simulink model "Project2"  (R2025b)
settings: Solver=VariableStepAuto  StartTime=0.0  StopTime=10  RelTol=1e-3
libraries: simulink x1
settings Model: Creator=night  LastModifiedBy=night

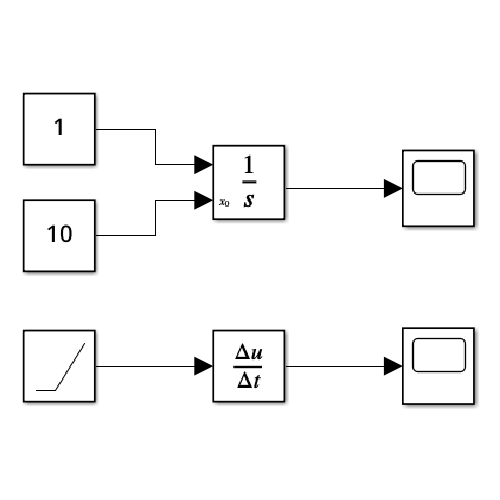
[thumbnail: Simulink's stored preview of the top-level diagram]
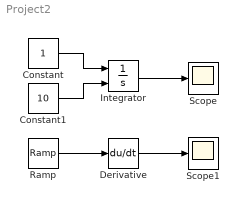
== system Project2 ==
  Constant : Constant
  Constant1 : Constant  Value=10
  Derivative : Derivative
  Integrator : Integrator  InitialConditionSource=external  InitialCondition=10
  Ramp : simulink/Sources/Ramp  slope=1  start=0  InitialOutput=0
  Scope : Scope
      settings: ActiveDisplayYMinimum=8.7500000000000036  ActiveDisplayYMaximum=21.249999999999964
  Scope1 : Scope
      settings: ActiveDisplayYMinimum=-0.12499999999999997  ActiveDisplayYMaximum=1.125
  wires:
  Constant/1 -> Integrator/1
  Integrator/1 -> Scope/1
  Derivative/1 -> Scope1/1
  Ramp/1 -> Derivative/1
  Constant1/1 -> Integrator/2
